simulink model "prey_predator"  (R2023b)
settings: Solver=VariableStepAuto  StartTime=0.0  StopTime=10.0  RelTol=1e-3
values from neighbouring files (symbols this model uses):
  a = 0.9    [prey_predator_script.m]
  b = 0.01    [prey_predator_script.m]
  c = 0.8    [prey_predator_script.m]
  d = 0.01    [prey_predator_script.m]
  x01 = 70    [prey_predator_script.m]
  x02 = 70    [prey_predator_script.m]
settings Model: Creator=martinhaugen  LastModifiedBy=martinhaugen

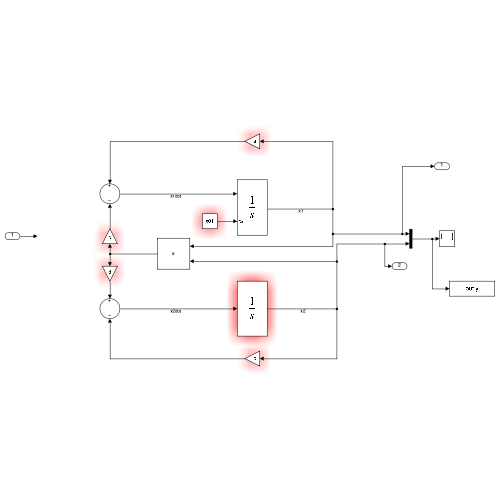
[thumbnail: Simulink's stored preview of the top-level diagram]
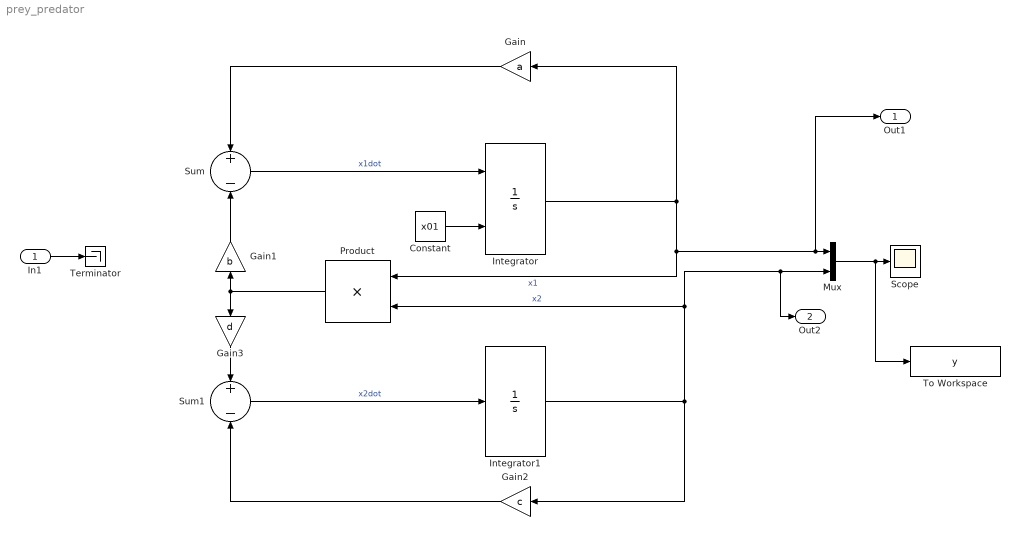
== system prey_predator ==
  In1 : Inport
  Constant : Constant  Value=x01
  Gain : Gain  Gain=a
  Gain1 : Gain  Gain=b
  Gain2 : Gain  Gain=c
  Gain3 : Gain  Gain=d
  Integrator : Integrator  InitialConditionSource=external
  Integrator1 : Integrator  InitialCondition=x02
  Mux : Mux  Inputs=2
  Product : Product
  Scope : Scope
  Sum : Sum  Inputs=+|-
  Sum1 : Sum  Inputs=+|-
  Terminator : Terminator
  To Workspace : ToWorkspace  VariableName=y  SaveFormat=Timeseries  SampleTime=-1
  Out1 : Outport
  Out2 : Outport  Port=2
  wires:
  Sum/1 -> Integrator/1  "x1dot"
  Integrator/1 -> Gain/1, Out1/1, Mux/1, Product/1  "x1"
  Gain/1 -> Sum/1
  Sum1/1 -> Integrator1/1  "x2dot"
  Integrator1/1 -> Out2/1, Mux/2, Product/2, Gain2/1  "x2"
  Gain1/1 -> Sum/2
  Product/1 -> Gain3/1, Gain1/1
  Gain2/1 -> Sum1/2
  Gain3/1 -> Sum1/1
  Mux/1 -> To Workspace/1, Scope/1
  Constant/1 -> Integrator/2
  In1/1 -> Terminator/1
